simulink model "FDScanningTool"  (R2022b)
settings: Solver=ode1  StartTime=0.0  StopTime=Tobs  FixedStep=delta_t  RelTol=1e-3
values from neighbouring files (symbols this model uses):
  C = 2*pi*Eo*inv(Rp)    [LineParameters.m]    (also in ParametrosAB.m = 2*pi*Epsilon*inv(P); exe_FDScanningTool.m = 0.001)
  delta_t = 10E-6    (= 1e-05)    [exe_FDScanningTool.m]
  dist_time = 1    [exe_FDScanningTool.m]
  dist_value_0 = Idist_value    (= 0.05)    [exe_FDScanningTool.m]
  dist_value_a = [Isignal_dist3(:,1),zeros(samples_window,1)]    [exe_FDScanningTool.m]
  dist_value_b = [Isignal_dist3(:,1),zeros(samples_window,1)]    [exe_FDScanningTool.m]
  dist_value_c = Isignal_dist3    [exe_FDScanningTool.m]
  dist_value_d = Idist_value    (= 0.05)    [exe_FDScanningTool.m]
  dist_value_n = 0.0    (= 0)    [exe_FDScanningTool.m]
  dist_value_p = 0.0    (= 0)    [exe_FDScanningTool.m]
  dist_value_q = 0.0    (= 0)    [exe_FDScanningTool.m]
  f0 = 50    [exe_FDScanningTool.m]    (also in multisine.m = fs/Ns)
  fd = fd0(n)    [exe_FDScanningTool.m]
  Ipeak = 1    [exe_FDScanningTool.m]
  L = 0.001    [exe_FDScanningTool.m]
  phi = (2/3)*pi    (= 2.09439510239)    [exe_FDScanningTool.m]
  R = cond1(:,6)    [LineParameters.m]    (also in exe_FDScanningTool.m = 0.01778)
  R_load = 1E-6    (= 1e-06)    [exe_FDScanningTool.m]
  Rsource = 1E-3    (= 0.001)    [exe_FDScanningTool.m]
  signal_type = 1    [exe_FDScanningTool.m]
  Vpeak = 1    [exe_FDScanningTool.m]
libraries: spsSeriesRLCBranchLib x21, spsControlledCurrentSourceLib x12, spsControlledVoltageSourceLib x12, spsThreePhaseVIMeasurementLib x10, spsThreePhaseSeriesRLCBranchLib x6, spsGroundLib x5, spsDistributedParametersLineFrequencyDependentLib x1, spspowerguiLib x1
(part 1 of 2)
settings Model: SimulationMode=accelerator  Creator=Luis Angel  LastModifiedBy=Luis Angel

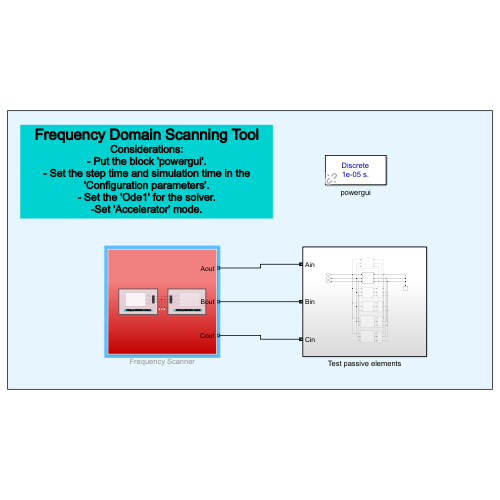
[thumbnail: Simulink's stored preview of the top-level diagram]
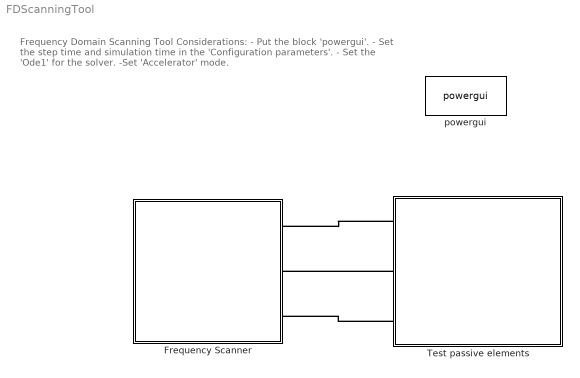
== system FDScanningTool ==
  note: Frequency Domain Scanning Tool
      | Considerations:
      | - Put the block 'powergui'.
      | - Set the step time and simulation time in the 'Configuration parameters'.
      | - Set the 'Ode1' for the solver.
      | -Set 'Accelerator' mode.
  Frequency Scanner : Subsystem
  Test passive elements : Subsystem
  powergui : spspowerguiLib/powergui  Priority=1  SimulationMode=Discrete  SampleTime=delta_t  frequency=60  Iterations=50  frequencyindice=0  Pbase=100e6  ErrMax=1e-4  UnitsV=kV  UnitsW=MW  buscounter=0  FunctionMessages=off  echomessages=off  EnableUseOfTLC=off  CurrentSourceSwitches=off  DisableSnubberDevices=off  DisableRonSwitches=off  DisableVfSwitches=off  DisplayEquations=off  AutomaticDiscreteSolvers=off  SolverType=Tustin/Backward Euler (TBE)  Interpol=off  ExternalGateDelay=off  methode=off  Ts=100  x0status=blocks  SPID=on  SwTol=0  HookPort=off  NonlinearTolerance=1e-4  nMaxIteration=100  ContinueOnMaxIteration=off  RestoreLinks=warning  ResistiveCurrentMeasurement=off  Frange=[0:2:500]  Ylog=off  Xlog=on  ShowGrid=off  save=off  variable=ZData  structure=0  ZoomFFT=off  StartTime=0.0  cycles=1  DisplayStyle=1  fundamental=60  FreqAxis=off  MaxFrequency=1000  frequencyindicesteady=1  RmsSteady=1  display=off
  connections:
  Test passive elements/LConn1 -- Frequency Scanner/RConn1
  Test passive elements/LConn2 -- Frequency Scanner/RConn2
  Test passive elements/LConn3 -- Frequency Scanner/RConn3

== system FDScanningTool/Frequency Scanner ==
  note: Current perturbation method
  note: Voltage perturbation method
  Current Strategy : Subsystem  Commented=on
  Three-Phase V-I Measurement1 : spsThreePhaseVIMeasurementLib/Three-Phase V-I Measurement  VoltageMeasurement=no  SetLabelV=on  LabelV=Vabc  Vpu=off  VpuLL=off  CurrentMeasurement=no  SetLabelI=on  LabelI=Iabc  Ipu=off  Pbase=100e6  Vbase=500e3  OutputType=Complex  PhasorSimulation=off  PSBequivalent=0
  Three-Phase V-I Measurement3 : spsThreePhaseVIMeasurementLib/Three-Phase V-I Measurement  VoltageMeasurement=no  SetLabelV=on  LabelV=Vabc  Vpu=off  VpuLL=off  CurrentMeasurement=no  SetLabelI=on  LabelI=Iabc  Ipu=off  Pbase=100e6  Vbase=500e3  OutputType=Complex  PhasorSimulation=off  PSBequivalent=0
  Voltage Strategy : Subsystem
  Aout : PMIOPort  Side=Right
  Bout : PMIOPort  Port=2  Side=Right
  Cout : PMIOPort  Port=3  Side=Right
  connections:
  Bout/RConn1 -- Three-Phase V-I Measurement3/RConn2 -- Three-Phase V-I Measurement1/RConn2
  Aout/RConn1 -- Three-Phase V-I Measurement3/RConn1 -- Three-Phase V-I Measurement1/RConn1
  Cout/RConn1 -- Three-Phase V-I Measurement1/RConn3 -- Three-Phase V-I Measurement3/RConn3
  Three-Phase V-I Measurement1/LConn1 -- Voltage Strategy/RConn1
  Three-Phase V-I Measurement1/LConn2 -- Voltage Strategy/RConn2
  Three-Phase V-I Measurement1/LConn3 -- Voltage Strategy/RConn3
  Three-Phase V-I Measurement3/LConn1 -- Current Strategy/LConn1
  Three-Phase V-I Measurement3/LConn2 -- Current Strategy/LConn2
  Three-Phase V-I Measurement3/LConn3 -- Current Strategy/LConn3

== system FDScanningTool/Test passive elements ==
  For the paper : spsDistributedParametersLineFrequencyDependentLib/Distributed Parameters Line (Frequency-Dependent)  Commented=on  WBfile=Line_735kV.mat  L=100  NbPhases=3  Frange=1.00e-02 Hz to 1.00e+05 Hz, 141 points.  Comments=|  Measurements=None
      | Example of a 735 KV three-phase line
      |
      | Three bundles of 4 Bersfort ACSR 1355 MCM conductors
      | Two 1/2 inch diameter steel grounds wires
      |
      | Ytower =Ymin =  average heights of conductors
      settings: LibrarySourceBlock=|
      | sps_lib/Power Grid Elements/Distributed Parameters Line
      | (Frequency-Dependent)
  Ground17 : spsGroundLib/Ground  LConnTagsString=a
  TL PI Asymmetrical : Subsystem  Commented=on
  TL PI Symmetrical : Subsystem  Commented=on
  Three-Phase Series RLC Branch1 : spsThreePhaseSeriesRLCBranchLib/Three-Phase Series RLC Branch  LConnTagsString=A|B|C  RConnTagsString=A|B|C  BranchType=RLC  Resistance=R  Inductance=L  Capacitance=C  Measurements=None
  Three-Phase Series RLC Branch11 : spsThreePhaseSeriesRLCBranchLib/Three-Phase Series RLC Branch  Commented=on  LConnTagsString=A|B|C  RConnTagsString=A|B|C  BranchType=R  Resistance=R_load  Inductance=1e-3  Capacitance=1e-6  Measurements=None
  Three-Phase Series RLC Branch12 : spsThreePhaseSeriesRLCBranchLib/Three-Phase Series RLC Branch  Commented=on  LConnTagsString=A|B|C  RConnTagsString=A|B|C  BranchType=R  Resistance=R_load  Inductance=1e-3  Capacitance=1e-6  Measurements=None
  Three-Phase Series RLC Branch2 : spsThreePhaseSeriesRLCBranchLib/Three-Phase Series RLC Branch  Commented=on  LConnTagsString=A|B|C  RConnTagsString=A|B|C  BranchType=R  Resistance=R_load  Inductance=1e-3  Capacitance=1e-6  Measurements=None
  Unbalanced RLC2 : Subsystem  Commented=on
  Ain : PMIOPort  Side=Left
  Bin : PMIOPort  Port=2  Side=Left
  Cin : PMIOPort  Port=3  Side=Left
  connections:
  TL PI Symmetrical/RConn1 -- Three-Phase Series RLC Branch11/LConn1
  Three-Phase Series RLC Branch12/LConn1 -- TL PI Asymmetrical/RConn1
  TL PI Symmetrical/LConn3 -- For the paper/LConn3 -- TL PI Asymmetrical/LConn3 -- Cin/RConn1 -- Unbalanced RLC2/LConn3 -- Three-Phase Series RLC Branch1/LConn3
  TL PI Asymmetrical/LConn1 -- For the paper/LConn1 -- Unbalanced RLC2/LConn1 -- Ain/RConn1 -- Three-Phase Series RLC Branch1/LConn1 -- TL PI Symmetrical/LConn1
  Three-Phase Series RLC Branch12/LConn2 -- TL PI Asymmetrical/RConn2
  Unbalanced RLC2/LConn2 -- For the paper/LConn2 -- TL PI Asymmetrical/LConn2 -- TL PI Symmetrical/LConn2 -- Bin/RConn1 -- Three-Phase Series RLC Branch1/LConn2
  TL PI Symmetrical/RConn2 -- Three-Phase Series RLC Branch11/LConn2
  Three-Phase Series RLC Branch12/LConn3 -- TL PI Asymmetrical/RConn3
  TL PI Symmetrical/RConn3 -- Three-Phase Series RLC Branch11/LConn3
  Three-Phase Series RLC Branch1/RConn2 -- Unbalanced RLC2/RConn2 -- Unbalanced RLC2/RConn3 -- Three-Phase Series RLC Branch1/RConn3 -- Three-Phase Series RLC Branch2/RConn3 -- Three-Phase Series RLC Branch12/RConn3 -- Three-Phase Series RLC Branch11/RConn3 -- Ground17/LConn1 -- Three-Phase Series RLC Branch2/RConn1 -- Three-Phase Series RLC Branch12/RConn1 -- Three-Phase Series RLC Branch11/RConn1 -- Unbalanced RLC2/RConn1 -- Three-Phase Series RLC Branch1/RConn1 -- Three-Phase Series RLC Branch2/RConn2 -- Three-Phase Series RLC Branch12/RConn2 -- Three-Phase Series RLC Branch11/RConn2
  For the paper/RConn1 -- Three-Phase Series RLC Branch2/LConn1
  For the paper/RConn2 -- Three-Phase Series RLC Branch2/LConn2
  For the paper/RConn3 -- Three-Phase Series RLC Branch2/LConn3

== system FDScanningTool/Frequency Scanner/Current Strategy ==
  note: qd0 scan
  note: Fundamental source
  note: pn0 scan
  note: ABC scan
  ABCdisturbance2 : Subsystem  Commented=on
  Current Fundamental Source : Subsystem
      settings: PortSchema="{\"entries\":[{\"content\":{\"sides\":[{\"content\":{\"connectorIds\":[\"Out1\"]},\"type\":\"ConnectorPlacement.EquallySpacedRectSide\",\"uuid\":\"2a4baa29-0316-4256-b4e1-e3ef1d370b3b\"},{\"content\":{\"connectorIds\":[\"RConn1\",\"RConn2\",\"RConn3\"],\"side\":\"RIGHT\"},\"type\":\"ConnectorPlacement.EquallySpacedRectSide\",\"uuid\":\"3108b85a-ac52-49ed-83a6-d77923640585\"},{\"content\":{\"connectorIds\":[],\"side\":\"TOP\"},\"type\":\"ConnectorPlacement.EquallySpacedRectSide\",\"uuid\":\"4093502e-3b8b-4232-aa57-5a461ca3ca63\"},{\"content\":{\"connectorIds\":[\"RConn4\"],\"side\":\"BOTTOM\"},\"type\":\"ConnectorPlacement.EquallySpacedRectSide\",\"uuid\":\"50c06102-7582-4746-a571-3f791f943454\"}]},\"type\":\"ConnectorPlacement.EquallySpacedConnector\",\"uuid\":\"209f4db4-fe77-48a5-84ae-6773984a343b\"}],\"packageUris\":[\"http://schema.mathworks.com/mf0/Connector/R2020b\"],\"version\":\"1.0\"}"
  Three-Phase V-I Measurement2 : spsThreePhaseVIMeasurementLib/Three-Phase V-I Measurement  VoltageMeasurement=no  SetLabelV=on  LabelV=Vabc  Vpu=off  VpuLL=off  CurrentMeasurement=no  SetLabelI=on  LabelI=Iabc  Ipu=off  Pbase=100e6  Vbase=500e3  OutputType=Complex  PhasorSimulation=off  PSBequivalent=0
  pn0disturbance2 : Subsystem
  qd0disturbance2 : Subsystem  Commented=on
      settings: PortSchema="{\"entries\":[{\"content\":{\"sides\":[{\"content\":{\"connectorIds\":[\"LConn1\",\"LConn2\",\"LConn3\",\"LConn4\"]},\"type\":\"ConnectorPlacement.EquallySpacedRectSide\",\"uuid\":\"96b61a08-e73c-4bf9-b44c-8e6d57b8ef4a\"},{\"content\":{\"connectorIds\":[\"RConn1\",\"RConn2\",\"RConn3\"],\"side\":\"RIGHT\"},\"type\":\"ConnectorPlacement.EquallySpacedRectSide\",\"uuid\":\"3a0e4222-9b60-4a58-9d08-3b159ebff1b9\"},{\"content\":{\"connectorIds\":[\"In1\"],\"side\":\"TOP\"},\"type\":\"ConnectorPlacement.EquallySpacedRectSide\",\"uuid\":\"61af63da-f353-4270-b8c9-89c35459604e\"}]},\"type\":\"ConnectorPlacement.EquallySpacedConnector\",\"uuid\":\"24d596f4-e3d4-42a2-b524-8b1140a91bdb\"}],\"packageUris\":[\"http://schema.mathworks.com/mf0/Connector/R2020b\"],\"version\":\"1.0\"}"
  Aout : PMIOPort  Side=Left
  Bout : PMIOPort  Port=2  Side=Left
  Cout : PMIOPort  Port=3  Side=Left
  wires:
  [theta] -> qd0disturbance2/1(theta)
  Current Fundamental Source/1(theta) -> [theta]
  connections:
  pn0disturbance2/RConn1 -- Aout/RConn1 -- ABCdisturbance2/RConn1 -- qd0disturbance2/RConn1
  pn0disturbance2/RConn2 -- Bout/RConn1 -- ABCdisturbance2/RConn2 -- qd0disturbance2/RConn2
  Current Fundamental Source/RConn2 -- Three-Phase V-I Measurement2/LConn2
  Three-Phase V-I Measurement2/RConn2 -- pn0disturbance2/LConn2 -- ABCdisturbance2/LConn2 -- qd0disturbance2/LConn2
  Current Fundamental Source/RConn3 -- Three-Phase V-I Measurement2/LConn3
  pn0disturbance2/RConn3 -- Cout/RConn1 -- ABCdisturbance2/RConn3 -- qd0disturbance2/RConn3
  Three-Phase V-I Measurement2/RConn1 -- pn0disturbance2/LConn1 -- ABCdisturbance2/LConn1 -- qd0disturbance2/LConn1
  Current Fundamental Source/RConn4 -- pn0disturbance2/LConn4 -- ABCdisturbance2/LConn4 -- qd0disturbance2/LConn4
  Three-Phase V-I Measurement2/RConn3 -- pn0disturbance2/LConn3 -- ABCdisturbance2/LConn3 -- qd0disturbance2/LConn3
  Current Fundamental Source/RConn1 -- Three-Phase V-I Measurement2/LConn1

== system FDScanningTool/Frequency Scanner/Voltage Strategy ==
  note: Fundamental source
  note: pn0 scan
  note: ABC scan
  note: qd0 scan
  ABCdisturbance : Subsystem  Commented=on
  Three-Phase V-I Measurement : spsThreePhaseVIMeasurementLib/Three-Phase V-I Measurement  VoltageMeasurement=no  SetLabelV=on  LabelV=Vabc  Vpu=off  VpuLL=off  CurrentMeasurement=no  SetLabelI=on  LabelI=Iabc  Ipu=off  Pbase=100e6  Vbase=500e3  OutputType=Complex  PhasorSimulation=off  PSBequivalent=0
  Voltage Fundamental Source : Subsystem
      settings: PortSchema="{\"entries\":[{\"content\":{\"sides\":[{\"content\":{\"connectorIds\":[\"Out1\"]},\"type\":\"ConnectorPlacement.EquallySpacedRectSide\",\"uuid\":\"3dbf8d23-22ab-4ddc-ae4a-19197e180312\"},{\"content\":{\"connectorIds\":[\"RConn1\",\"RConn2\",\"RConn3\"],\"side\":\"RIGHT\"},\"type\":\"ConnectorPlacement.EquallySpacedRectSide\",\"uuid\":\"df914263-db35-4888-aa99-5dec7a54c6e0\"},{\"content\":{\"connectorIds\":[],\"side\":\"TOP\"},\"type\":\"ConnectorPlacement.EquallySpacedRectSide\",\"uuid\":\"815bd59d-9d4f-4637-8c0a-95368e7d07f9\"}]},\"type\":\"ConnectorPlacement.EquallySpacedConnector\",\"uuid\":\"b7ffca83-a6f6-4340-8cfa-6aec16cec0d1\"}],\"packageUris\":[\"http://schema.mathworks.com/mf0/Connector/R2020b\"],\"version\":\"1.0\"}"
  pn0disturbance : Subsystem
  qd0disturbance : Subsystem  Commented=on
      settings: PortSchema="{\"entries\":[{\"content\":{\"sides\":[{\"content\":{\"connectorIds\":[\"LConn1\",\"LConn2\",\"LConn3\"]},\"type\":\"ConnectorPlacement.EquallySpacedRectSide\",\"uuid\":\"96b61a08-e73c-4bf9-b44c-8e6d57b8ef4a\"},{\"content\":{\"connectorIds\":[\"RConn1\",\"RConn2\",\"RConn3\"],\"side\":\"RIGHT\"},\"type\":\"ConnectorPlacement.EquallySpacedRectSide\",\"uuid\":\"3a0e4222-9b60-4a58-9d08-3b159ebff1b9\"},{\"content\":{\"connectorIds\":[\"In1\"],\"side\":\"TOP\"},\"type\":\"ConnectorPlacement.EquallySpacedRectSide\",\"uuid\":\"61af63da-f353-4270-b8c9-89c35459604e\"}]},\"type\":\"ConnectorPlacement.EquallySpacedConnector\",\"uuid\":\"24d596f4-e3d4-42a2-b524-8b1140a91bdb\"}],\"packageUris\":[\"http://schema.mathworks.com/mf0/Connector/R2020b\"],\"version\":\"1.0\"}"
  Aout : PMIOPort  Side=Right
  Bout : PMIOPort  Port=2  Side=Right
  Cout : PMIOPort  Port=3  Side=Right
  wires:
  Voltage Fundamental Source/1(theta) -> [theta]
  [theta] -> qd0disturbance/1(theta)
  connections:
  ABCdisturbance/RConn2 -- Bout/RConn1 -- pn0disturbance/RConn2 -- qd0disturbance/RConn2
  Voltage Fundamental Source/RConn1 -- Three-Phase V-I Measurement/LConn1
  qd0disturbance/LConn3 -- ABCdisturbance/LConn3 -- Three-Phase V-I Measurement/RConn3 -- pn0disturbance/LConn3
  ABCdisturbance/RConn1 -- Aout/RConn1 -- pn0disturbance/RConn1 -- qd0disturbance/RConn1
  Voltage Fundamental Source/RConn2 -- Three-Phase V-I Measurement/LConn2
  Voltage Fundamental Source/RConn3 -- Three-Phase V-I Measurement/LConn3
  ABCdisturbance/RConn3 -- Cout/RConn1 -- pn0disturbance/RConn3 -- qd0disturbance/RConn3
  qd0disturbance/LConn1 -- ABCdisturbance/LConn1 -- Three-Phase V-I Measurement/RConn1 -- pn0disturbance/LConn1
  qd0disturbance/LConn2 -- ABCdisturbance/LConn2 -- Three-Phase V-I Measurement/RConn2 -- pn0disturbance/LConn2

== system FDScanningTool/Test passive elements/TL PI Asymmetrical ==
  Ground6 : spsGroundLib/Ground  LConnTagsString=a
  Series RLC Branch1 : spsSeriesRLCBranchLib/Series RLC Branch  LConnTagsString=__new0  RConnTagsString=__new0  BranchType=RL  Resistance=R*0.9  Inductance=L*0.9  SetiL0=off  InitialCurrent=0  Capacitance=1e-6  Setx0=off  InitialVoltage=0  Measurements=None
  Series RLC Branch2 : spsSeriesRLCBranchLib/Series RLC Branch  LConnTagsString=__new0  RConnTagsString=__new0  BranchType=C  Resistance=1  Inductance=1e-3  SetiL0=off  InitialCurrent=0  Capacitance=C*0.9/2  Setx0=off  InitialVoltage=Vinit  Measurements=None
  Series RLC Branch3 : spsSeriesRLCBranchLib/Series RLC Branch  LConnTagsString=__new0  RConnTagsString=__new0  BranchType=RL  Resistance=R  Inductance=L  SetiL0=off  InitialCurrent=0  Capacitance=1e-6  Setx0=off  InitialVoltage=0  Measurements=None
  Series RLC Branch4 : spsSeriesRLCBranchLib/Series RLC Branch  LConnTagsString=__new0  RConnTagsString=__new0  BranchType=C  Resistance=1  Inductance=1e-3  SetiL0=off  InitialCurrent=0  Capacitance=C/2  Setx0=off  InitialVoltage=Vinit  Measurements=None
  Series RLC Branch5 : spsSeriesRLCBranchLib/Series RLC Branch  LConnTagsString=__new0  RConnTagsString=__new0  BranchType=C  Resistance=1  Inductance=1e-3  SetiL0=off  InitialCurrent=0  Capacitance=C/2  Setx0=off  InitialVoltage=Vinit  Measurements=None
  Series RLC Branch6 : spsSeriesRLCBranchLib/Series RLC Branch  LConnTagsString=__new0  RConnTagsString=__new0  BranchType=C  Resistance=1  Inductance=1e-3  SetiL0=off  InitialCurrent=0  Capacitance=C*0.9/2  Setx0=off  InitialVoltage=Vinit  Measurements=None
  Series RLC Branch7 : spsSeriesRLCBranchLib/Series RLC Branch  LConnTagsString=__new0  RConnTagsString=__new0  BranchType=RL  Resistance=R*0.8  Inductance=L*0.8  SetiL0=off  InitialCurrent=0  Capacitance=1e-6  Setx0=off  InitialVoltage=0  Measurements=None
  Series RLC Branch8 : spsSeriesRLCBranchLib/Series RLC Branch  LConnTagsString=__new0  RConnTagsString=__new0  BranchType=C  Resistance=1  Inductance=1e-3  SetiL0=off  InitialCurrent=0  Capacitance=C*0.8/2  Setx0=off  InitialVoltage=Vinit  Measurements=None
  Series RLC Branch9 : spsSeriesRLCBranchLib/Series RLC Branch  LConnTagsString=__new0  RConnTagsString=__new0  BranchType=C  Resistance=1  Inductance=1e-3  SetiL0=off  InitialCurrent=0  Capacitance=C*0.8/2  Setx0=off  InitialVoltage=Vinit  Measurements=None
  A : PMIOPort  Side=Left
  B : PMIOPort  Port=2  Side=Left
  C : PMIOPort  Port=3  Side=Left
  a : PMIOPort  Port=4  Side=Right
  b : PMIOPort  Port=5  Side=Right
  c : PMIOPort  Port=6  Side=Right
  connections:
  Series RLC Branch5/LConn1 -- a/RConn1 -- Series RLC Branch3/RConn1
  Series RLC Branch2/RConn1 -- Series RLC Branch6/RConn1 -- Series RLC Branch8/RConn1 -- Series RLC Branch9/RConn1 -- Ground6/LConn1 -- Series RLC Branch5/RConn1 -- Series RLC Branch4/RConn1
  Series RLC Branch3/LConn1 -- A/RConn1 -- Series RLC Branch4/LConn1
  Series RLC Branch1/LConn1 -- Series RLC Branch2/LConn1 -- B/RConn1
  Series RLC Branch6/LConn1 -- Series RLC Branch1/RConn1 -- b/RConn1
  Series RLC Branch7/LConn1 -- Series RLC Branch8/LConn1 -- C/RConn1
  Series RLC Branch9/LConn1 -- Series RLC Branch7/RConn1 -- c/RConn1

== system FDScanningTool/Test passive elements/TL PI Symmetrical ==
  Ground3 : spsGroundLib/Ground  LConnTagsString=a
  Series RLC Branch1 : spsSeriesRLCBranchLib/Series RLC Branch  LConnTagsString=__new0  RConnTagsString=__new0  BranchType=RL  Resistance=R  Inductance=L  SetiL0=off  InitialCurrent=0  Capacitance=1e-6  Setx0=off  InitialVoltage=0  Measurements=None
  Series RLC Branch{2,4..6,8..9} (6 alike) : spsSeriesRLCBranchLib/Series RLC Branch  LConnTagsString=__new0  RConnTagsString=__new0  BranchType=C  Resistance=1  Inductance=1e-3  SetiL0=off  InitialCurrent=0  Capacitance=C/2  Setx0=off  InitialVoltage=Vinit  Measurements=None
  Series RLC Branch3 : spsSeriesRLCBranchLib/Series RLC Branch  LConnTagsString=__new0  RConnTagsString=__new0  BranchType=RL  Resistance=R  Inductance=L  SetiL0=off  InitialCurrent=0  Capacitance=1e-6  Setx0=off  InitialVoltage=0  Measurements=None
  Series RLC Branch7 : spsSeriesRLCBranchLib/Series RLC Branch  LConnTagsString=__new0  RConnTagsString=__new0  BranchType=RL  Resistance=R  Inductance=L  SetiL0=off  InitialCurrent=0  Capacitance=1e-6  Setx0=off  InitialVoltage=0  Measurements=None
  A : PMIOPort  Side=Left
  B : PMIOPort  Port=2  Side=Left
  C : PMIOPort  Port=3  Side=Left
  a : PMIOPort  Port=4  Side=Right
  b : PMIOPort  Port=5  Side=Right
  c : PMIOPort  Port=6  Side=Right
  connections:
  Series RLC Branch5/LConn1 -- a/RConn1 -- Series RLC Branch3/RConn1
  Series RLC Branch3/LConn1 -- A/RConn1 -- Series RLC Branch4/LConn1
  Series RLC Branch1/LConn1 -- Series RLC Branch2/LConn1 -- B/RConn1
  Series RLC Branch6/LConn1 -- Series RLC Branch1/RConn1 -- b/RConn1
  Series RLC Branch6/RConn1 -- Series RLC Branch8/RConn1 -- Series RLC Branch9/RConn1 -- Series RLC Branch4/RConn1 -- Series RLC Branch5/RConn1 -- Ground3/LConn1 -- Series RLC Branch2/RConn1
  Series RLC Branch7/LConn1 -- Series RLC Branch8/LConn1 -- C/RConn1
  Series RLC Branch9/LConn1 -- Series RLC Branch7/RConn1 -- c/RConn1

== system FDScanningTool/Test passive elements/Unbalanced RLC2 ==
  Series RLC Branch : spsSeriesRLCBranchLib/Series RLC Branch  LConnTagsString=__new0  RConnTagsString=__new0  BranchType=RLC  Resistance=R  Inductance=L  SetiL0=off  InitialCurrent=0  Capacitance=C  Setx0=off  InitialVoltage=0  Measurements=None
  Series RLC Branch1 : spsSeriesRLCBranchLib/Series RLC Branch  LConnTagsString=__new0  RConnTagsString=__new0  BranchType=RLC  Resistance=R*0.9  Inductance=L*0.9  SetiL0=off  InitialCurrent=0  Capacitance=C*0.9  Setx0=off  InitialVoltage=0  Measurements=None
  Series RLC Branch2 : spsSeriesRLCBranchLib/Series RLC Branch  LConnTagsString=__new0  RConnTagsString=__new0  BranchType=RLC  Resistance=R*0.8  Inductance=L*0.8  SetiL0=off  InitialCurrent=0  Capacitance=C*0.8  Setx0=off  InitialVoltage=0  Measurements=None
  Conn1 : PMIOPort  Side=Left
  Conn2 : PMIOPort  Port=2  Side=Right
  Conn3 : PMIOPort  Port=3  Side=Left
  Conn4 : PMIOPort  Port=4  Side=Right
  Conn5 : PMIOPort  Port=5  Side=Left
  Conn6 : PMIOPort  Port=6  Side=Right
  connections:
  Series RLC Branch/LConn1 -- Conn1/RConn1
  Series RLC Branch2/RConn1 -- Conn6/RConn1
  Series RLC Branch1/RConn1 -- Conn4/RConn1
  Series RLC Branch2/LConn1 -- Conn5/RConn1
  Series RLC Branch1/LConn1 -- Conn3/RConn1
  Series RLC Branch/RConn1 -- Conn2/RConn1

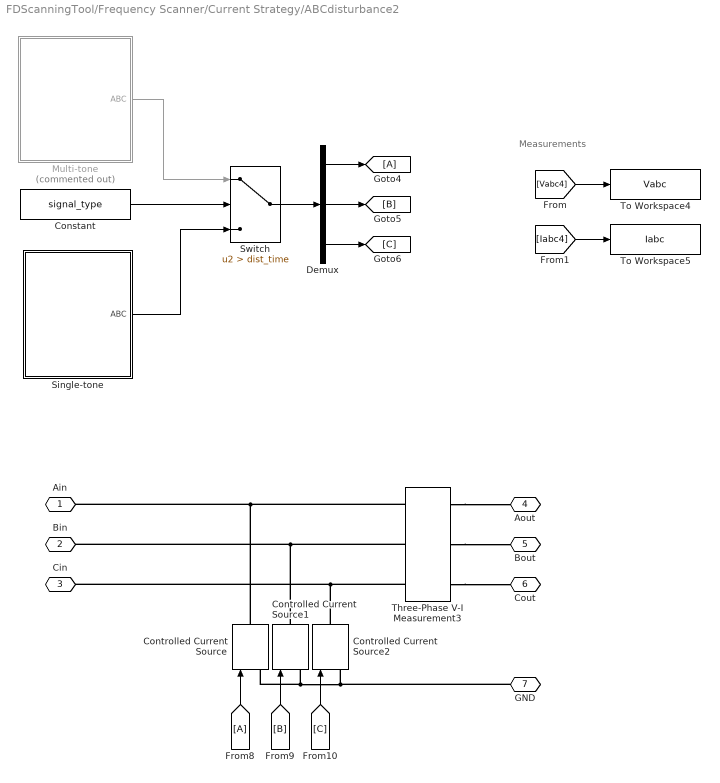
== system FDScanningTool/Frequency Scanner/Current Strategy/ABCdisturbance2 ==
  note: Measurements
  Constant : Constant  Value=signal_type
  Controlled Current Source : spsControlledCurrentSourceLib/Controlled Current Source  Initialize=off  Source_Type=AC  Amplitude=0  Phase=0  Frequency=0  Measurements=None
  Controlled Current Source1 : spsControlledCurrentSourceLib/Controlled Current Source  Initialize=off  Source_Type=AC  Amplitude=0  Phase=0  Frequency=0  Measurements=None
  Controlled Current Source2 : spsControlledCurrentSourceLib/Controlled Current Source  Initialize=off  Source_Type=AC  Amplitude=0  Phase=0  Frequency=0  Measurements=None
  Demux : Demux  Outputs=3
  From8 : From
  Goto4 : Goto
  Multi-tone : Subsystem  Commented=on
  Single-tone : Subsystem
  Switch : Switch  Criteria=u2 > Threshold  Threshold=dist_time  SaturateOnIntegerOverflow=off  InputSameDT=off
  Three-Phase V-I Measurement3 : spsThreePhaseVIMeasurementLib/Three-Phase V-I Measurement  VoltageMeasurement=phase-to-ground  SetLabelV=on  LabelV=Vabc4  Vpu=off  VpuLL=off  CurrentMeasurement=yes  SetLabelI=on  LabelI=Iabc4  Ipu=off  Pbase=100e6  Vbase=500e3  OutputType=Complex  PhasorSimulation=off  PSBequivalent=0
  To Workspace4 : ToWorkspace  VariableName=Vabc  SampleTime=-1
  To Workspace5 : ToWorkspace  VariableName=Iabc  SampleTime=-1
  Ain : PMIOPort  Side=Left
  Bin : PMIOPort  Port=2  Side=Left
  Cin : PMIOPort  Port=3  Side=Left
  Aout : PMIOPort  Port=4  Side=Right
  Bout : PMIOPort  Port=5  Side=Right
  Cout : PMIOPort  Port=6  Side=Right
  GND : PMIOPort  Port=7  Side=Left
  wires:
  [Vabc4] -> To Workspace4/1
  [Iabc4] -> To Workspace5/1
  [C] -> Controlled Current Source2/1
  [B] -> Controlled Current Source1/1
  From8/1 -> Controlled Current Source/1
  Constant/1 -> Switch/2
  Multi-tone/1(ABC) -> Switch/1
  Demux/1 -> Goto4/1
  Demux/2 -> [B]
  Demux/3 -> [C]
  Switch/1 -> Demux/1
  Single-tone/1(ABC) -> Switch/3
  connections:
  Controlled Current Source1/LConn1 -- GND/RConn1 -- Controlled Current Source2/LConn1 -- Controlled Current Source/LConn1
  Controlled Current Source/RConn1 -- Three-Phase V-I Measurement3/LConn1 -- Ain/RConn1
  Controlled Current Source2/RConn1 -- Three-Phase V-I Measurement3/LConn3 -- Cin/RConn1
  Controlled Current Source1/RConn1 -- Three-Phase V-I Measurement3/LConn2 -- Bin/RConn1
  Three-Phase V-I Measurement3/RConn1 -- Aout/RConn1
  Three-Phase V-I Measurement3/RConn2 -- Bout/RConn1
  Three-Phase V-I Measurement3/RConn3 -- Cout/RConn1

== system FDScanningTool/Frequency Scanner/Current Strategy/Current Fundamental Source ==
  Controlled Current Source : spsControlledCurrentSourceLib/Controlled Current Source  Initialize=off  Source_Type=AC  Amplitude=0  Phase=0  Frequency=0  Measurements=None
  Controlled Current Source1 : spsControlledCurrentSourceLib/Controlled Current Source  Initialize=off  Source_Type=AC  Amplitude=0  Phase=0  Frequency=0  Measurements=None
  Controlled Current Source2 : spsControlledCurrentSourceLib/Controlled Current Source  Initialize=off  Source_Type=AC  Amplitude=0  Phase=0  Frequency=0  Measurements=None
  Grid Voltages1 : Subsystem
  Ground : spsGroundLib/Ground  LConnTagsString=a
  Three-Phase Series RLC Branch : spsThreePhaseSeriesRLCBranchLib/Three-Phase Series RLC Branch  LConnTagsString=A|B|C  RConnTagsString=A|B|C  BranchType=R  Resistance=1/Rsource  Inductance=1e-3  Capacitance=1e-6  Measurements=None
  VzA : PMIOPort  Side=Right
  VzB : PMIOPort  Port=2  Side=Right
  VzC : PMIOPort  Port=3  Side=Right
  GND : PMIOPort  Port=4  Side=Right
  theta : Outport
  wires:
  Grid Voltages1/3(VC) -> Controlled Current Source/1
  Grid Voltages1/2(VB) -> Controlled Current Source1/1
  Grid Voltages1/1(VA) -> Controlled Current Source2/1
  Grid Voltages1/4(theta) -> theta/1
  connections:
  Controlled Current Source2/RConn1 -- Three-Phase Series RLC Branch/LConn1 -- VzA/RConn1
  Controlled Current Source1/RConn1 -- Three-Phase Series RLC Branch/LConn2 -- VzB/RConn1
  Controlled Current Source/RConn1 -- Three-Phase Series RLC Branch/LConn3 -- VzC/RConn1
  Ground/LConn1 -- Controlled Current Source/LConn1 -- Controlled Current Source1/LConn1 -- Controlled Current Source2/LConn1 -- Three-Phase Series RLC Branch/RConn3 -- Three-Phase Series RLC Branch/RConn2 -- Three-Phase Series RLC Branch/RConn1 -- GND/RConn1

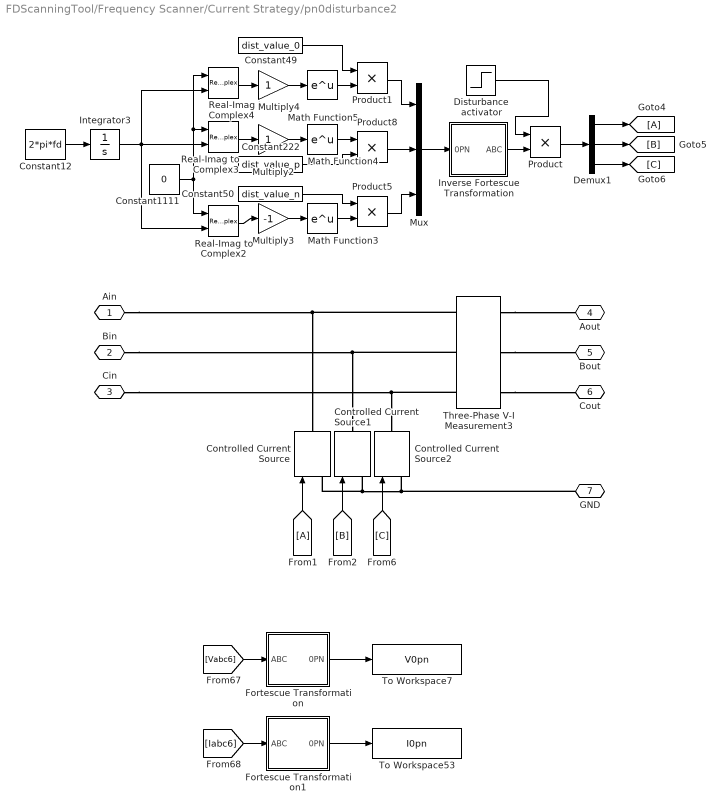
== system FDScanningTool/Frequency Scanner/Current Strategy/pn0disturbance2 ==
  Constant1111 : Constant  Value=0
  Constant12 : Constant  Value=2*pi*fd  SampleTime=delta_t
  Constant222 : Constant  Value=dist_value_p
  Constant49 : Constant  Value=dist_value_0
  Constant50 : Constant  Value=dist_value_n
  Controlled Current Source : spsControlledCurrentSourceLib/Controlled Current Source  Initialize=off  Source_Type=AC  Amplitude=0  Phase=0  Frequency=0  Measurements=None
  Controlled Current Source1 : spsControlledCurrentSourceLib/Controlled Current Source  Initialize=off  Source_Type=AC  Amplitude=0  Phase=0  Frequency=0  Measurements=None
  Controlled Current Source2 : spsControlledCurrentSourceLib/Controlled Current Source  Initialize=off  Source_Type=AC  Amplitude=0  Phase=0  Frequency=0  Measurements=None
  Demux1 : Demux  Outputs=3
  Disturbance activator : Step  Time=dist_time  SampleTime=delta_t
  Fortescue Transformation : Subsystem
  Fortescue Transformation1 : Subsystem
  From1 : From
  Goto4 : Goto
  Integrator3 : Integrator
  Inverse Fortescue Transformation : Subsystem
  Math Function3 : Math
  Math Function4 : Math
  Math Function5 : Math
  Multiply2 : Gain
  Multiply3 : Gain  Gain=-1
  Multiply4 : Gain
  Mux : Mux  Inputs=3
  Product{,1,5,8} (4 alike) : Product
  Real-Imag to Complex2 : RealImagToComplex
  Real-Imag to Complex3 : RealImagToComplex
  Real-Imag to Complex4 : RealImagToComplex
  Three-Phase V-I Measurement3 : spsThreePhaseVIMeasurementLib/Three-Phase V-I Measurement  VoltageMeasurement=phase-to-ground  SetLabelV=on  LabelV=Vabc6  Vpu=off  VpuLL=off  CurrentMeasurement=yes  SetLabelI=on  LabelI=Iabc6  Ipu=off  Pbase=100e6  Vbase=500e3  OutputType=Complex  PhasorSimulation=off  PSBequivalent=0
  To Workspace53 : ToWorkspace  VariableName=I0pn  SampleTime=-1
  To Workspace7 : ToWorkspace  VariableName=V0pn  SampleTime=-1
  Ain : PMIOPort  Side=Left
  Bin : PMIOPort  Port=2  Side=Left
  Cin : PMIOPort  Port=3  Side=Left
  Aout : PMIOPort  Port=4  Side=Right
  Bout : PMIOPort  Port=5  Side=Right
  Cout : PMIOPort  Port=6  Side=Right
  GND : PMIOPort  Port=7  Side=Left
  wires:
  Product/1 -> Demux1/1
  Demux1/1 -> Goto4/1
  Demux1/3 -> [C]
  Demux1/2 -> [B]
  Mux/1 -> Inverse Fortescue Transformation/1(0PN)
  Multiply2/1 -> Math Function4/1
  Integrator3/1 -> Real-Imag to Complex2/2, Real-Imag to Complex3/2, Real-Imag to Complex4/2
  Constant1111/1 -> Real-Imag to Complex4/1, Real-Imag to Complex3/1, Real-Imag to Complex2/1
  Real-Imag to Complex3/1 -> Multiply2/1
  Multiply3/1 -> Math Function3/1
  Constant12/1 -> Integrator3/1
  Real-Imag to Complex2/1 -> Multiply3/1
  Math Function5/1 -> Product1/2
  Real-Imag to Complex4/1 -> Multiply4/1
  Multiply4/1 -> Math Function5/1
  Product1/1 -> Mux/1
  Disturbance activator/1 -> Product/1
  Inverse Fortescue Transformation/1(ABC) -> Product/2
  Constant49/1 -> Product1/1
  Math Function3/1 -> Product5/2
  Constant50/1 -> Product5/1
  Math Function4/1 -> Product8/1
  Constant222/1 -> Product8/2
  Product8/1 -> Mux/2
  Product5/1 -> Mux/3
  [Vabc6] -> Fortescue Transformation/1(ABC)
  [Iabc6] -> Fortescue Transformation1/1(ABC)
  Fortescue Transformation/1(0PN) -> To Workspace7/1
  Fortescue Transformation1/1(0PN) -> To Workspace53/1
  [B] -> Controlled Current Source1/1
  [C] -> Controlled Current Source2/1
  From1/1 -> Controlled Current Source/1
  connections:
  Cin/RConn1 -- Three-Phase V-I Measurement3/LConn3 -- Controlled Current Source2/RConn1
  Controlled Current Source1/LConn1 -- GND/RConn1 -- Controlled Current Source2/LConn1 -- Controlled Current Source/LConn1
  Ain/RConn1 -- Three-Phase V-I Measurement3/LConn1 -- Controlled Current Source/RConn1
  Bin/RConn1 -- Three-Phase V-I Measurement3/LConn2 -- Controlled Current Source1/RConn1
  Three-Phase V-I Measurement3/RConn3 -- Cout/RConn1
  Three-Phase V-I Measurement3/RConn2 -- Bout/RConn1
  Three-Phase V-I Measurement3/RConn1 -- Aout/RConn1

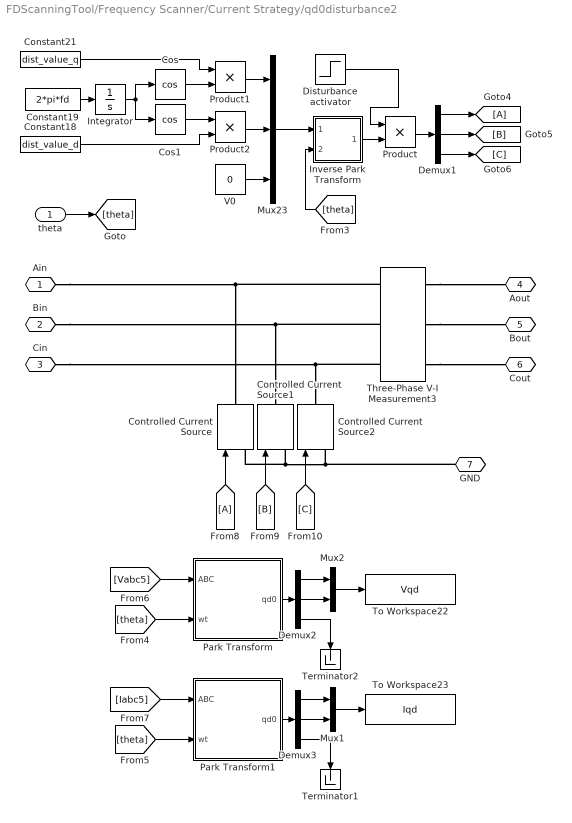
== system FDScanningTool/Frequency Scanner/Current Strategy/qd0disturbance2 ==
  theta : Inport
  Constant18 : Constant  Value=dist_value_d
  Constant19 : Constant  Value=2*pi*fd
  Constant21 : Constant  Value=dist_value_q
  Controlled Current Source : spsControlledCurrentSourceLib/Controlled Current Source  Initialize=off  Source_Type=AC  Amplitude=0  Phase=0  Frequency=0  Measurements=None
  Controlled Current Source1 : spsControlledCurrentSourceLib/Controlled Current Source  Initialize=off  Source_Type=AC  Amplitude=0  Phase=0  Frequency=0  Measurements=None
  Controlled Current Source2 : spsControlledCurrentSourceLib/Controlled Current Source  Initialize=off  Source_Type=AC  Amplitude=0  Phase=0  Frequency=0  Measurements=None
  Cos : Trigonometry  Operator=cos
  Cos1 : Trigonometry  Operator=cos
  Demux1 : Demux  Outputs=3
  Demux2 : Demux  Outputs=3
  Demux3 : Demux  Outputs=3
  Disturbance activator : Step  Time=dist_time  Before=0.0  After=1.0  SampleTime=delta_t
  From8 : From
  Goto4 : Goto
  Integrator : Integrator
  Inverse Park Transform : Subsystem
  Mux1 : Mux  Inputs=2
  Mux2 : Mux  Inputs=2
  Mux23 : Mux  Inputs=3
  Park Transform : Subsystem
  Park Transform1 : Subsystem
  Product : Product
  Product1 : Product
  Product2 : Product
  Terminator1 : Terminator
  Terminator2 : Terminator
  Three-Phase V-I Measurement3 : spsThreePhaseVIMeasurementLib/Three-Phase V-I Measurement  VoltageMeasurement=phase-to-ground  SetLabelV=on  LabelV=Vabc5  Vpu=off  VpuLL=off  CurrentMeasurement=yes  SetLabelI=on  LabelI=Iabc5  Ipu=off  Pbase=100e6  Vbase=500e3  OutputType=Complex  PhasorSimulation=off  PSBequivalent=0
  To Workspace22 : ToWorkspace  VariableName=Vqd  SampleTime=-1
  To Workspace23 : ToWorkspace  VariableName=Iqd  SampleTime=-1
  V0 : Constant  Value=0
  Ain : PMIOPort  Side=Left
  Bin : PMIOPort  Port=2  Side=Left
  Cin : PMIOPort  Port=3  Side=Left
  Aout : PMIOPort  Port=4  Side=Right
  Bout : PMIOPort  Port=5  Side=Right
  Cout : PMIOPort  Port=6  Side=Right
  GND : PMIOPort  Port=7  Side=Left
  wires:
  Mux23/1 -> Inverse Park Transform/1(qd0)
  V0/1 -> Mux23/3
  Product/1 -> Demux1/1
  Demux1/1 -> Goto4/1
  Demux1/3 -> [C]
  Demux1/2 -> [B]
  Cos/1 -> Product1/2
  Constant21/1 -> Product1/1
  Product1/1 -> Mux23/1
  Cos1/1 -> Product2/1
  Integrator/1 -> Cos/1, Cos1/1
  Constant19/1 -> Integrator/1
  Product2/1 -> Mux23/2
  Constant18/1 -> Product2/2
  Mux2/1 -> To Workspace22/1
  [theta] -> Park Transform/2(wt)
  [Vabc5] -> Park Transform/1(ABC)
  Park Transform/1(qd0) -> Demux2/1
  Demux2/3 -> Terminator2/1
  theta/1 -> [theta]
  [theta] -> Inverse Park Transform/2(theta)
  Inverse Park Transform/1(ABC) -> Product/2
  Disturbance activator/1 -> Product/1
  Demux2/1 -> Mux2/1
  Demux2/2 -> Mux2/2
  Mux1/1 -> To Workspace23/1
  Demux3/3 -> Terminator1/1
  [Iabc5] -> Park Transform1/1(ABC)
  Park Transform1/1(qd0) -> Demux3/1
  Demux3/2 -> Mux1/2
  Demux3/1 -> Mux1/1
  [theta] -> Park Transform1/2(wt)
  From8/1 -> Controlled Current Source/1
  [C] -> Controlled Current Source2/1
  [B] -> Controlled Current Source1/1
  connections:
  Controlled Current Source1/LConn1 -- GND/RConn1 -- Controlled Current Source2/LConn1 -- Controlled Current Source/LConn1
  Ain/RConn1 -- Three-Phase V-I Measurement3/LConn1 -- Controlled Current Source/RConn1
  Bin/RConn1 -- Three-Phase V-I Measurement3/LConn2 -- Controlled Current Source1/RConn1
  Cin/RConn1 -- Three-Phase V-I Measurement3/LConn3 -- Controlled Current Source2/RConn1
  Three-Phase V-I Measurement3/RConn1 -- Aout/RConn1
  Three-Phase V-I Measurement3/RConn2 -- Bout/RConn1
  Three-Phase V-I Measurement3/RConn3 -- Cout/RConn1

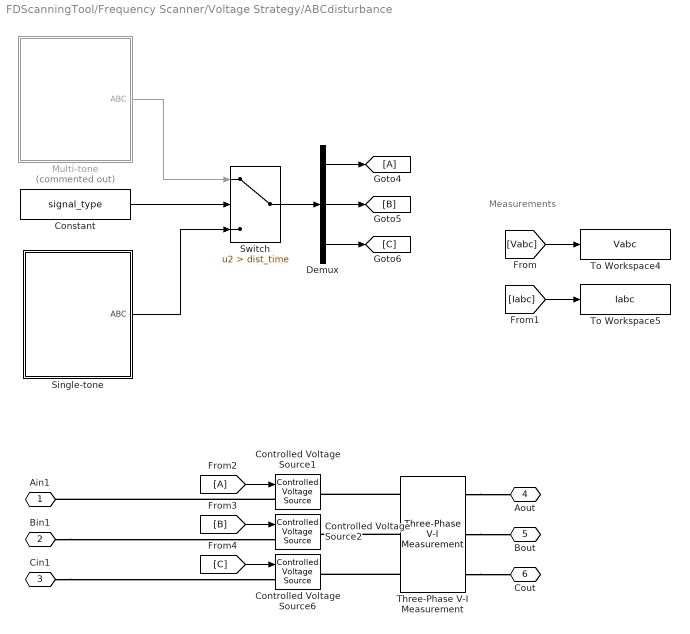
== system FDScanningTool/Frequency Scanner/Voltage Strategy/ABCdisturbance ==
  note: Measurements
  Constant : Constant  Value=signal_type
  Controlled Voltage Source1 : spsControlledVoltageSourceLib/Controlled Voltage Source  Initialize=off  Source_Type=DC  Amplitude=0  Phase=0  Frequency=0  Measurements=None
  Controlled Voltage Source2 : spsControlledVoltageSourceLib/Controlled Voltage Source  Initialize=off  Source_Type=DC  Amplitude=0  Phase=0  Frequency=0  Measurements=None
  Controlled Voltage Source6 : spsControlledVoltageSourceLib/Controlled Voltage Source  Initialize=off  Source_Type=DC  Amplitude=0  Phase=0  Frequency=0  Measurements=None
  Demux : Demux  Outputs=3
  From2 : From
  Goto4 : Goto
  Multi-tone : Subsystem  Commented=on
  Single-tone : Subsystem
  Switch : Switch  Criteria=u2 > Threshold  Threshold=dist_time  SaturateOnIntegerOverflow=off  InputSameDT=off
  Three-Phase V-I Measurement : spsThreePhaseVIMeasurementLib/Three-Phase V-I Measurement  VoltageMeasurement=phase-to-ground  SetLabelV=on  LabelV=Vabc  Vpu=off  VpuLL=off  CurrentMeasurement=yes  SetLabelI=on  LabelI=Iabc  Ipu=off  Pbase=100e6  Vbase=500e3  OutputType=Complex  PhasorSimulation=off  PSBequivalent=0
  To Workspace4 : ToWorkspace  VariableName=Vabc  SampleTime=-1
  To Workspace5 : ToWorkspace  VariableName=Iabc  SampleTime=-1
  Ain1 : PMIOPort  Side=Left
  Bin1 : PMIOPort  Port=2  Side=Left
  Cin1 : PMIOPort  Port=3  Side=Left
  Aout : PMIOPort  Port=4  Side=Right
  Bout : PMIOPort  Port=5  Side=Right
  Cout : PMIOPort  Port=6  Side=Right
  wires:
  [Vabc] -> To Workspace4/1
  [Iabc] -> To Workspace5/1
  [C] -> Controlled Voltage Source6/1
  From2/1 -> Controlled Voltage Source1/1
  [B] -> Controlled Voltage Source2/1
  Multi-tone/1(ABC) -> Switch/1
  Demux/3 -> [C]
  Constant/1 -> Switch/2
  Demux/1 -> Goto4/1
  Demux/2 -> [B]
  Single-tone/1(ABC) -> Switch/3
  Switch/1 -> Demux/1
  connections:
  Bin1/RConn1 -- Controlled Voltage Source2/LConn1
  Controlled Voltage Source1/LConn1 -- Ain1/RConn1
  Cin1/RConn1 -- Controlled Voltage Source6/LConn1
  Three-Phase V-I Measurement/LConn1 -- Controlled Voltage Source1/RConn1
  Three-Phase V-I Measurement/LConn2 -- Controlled Voltage Source2/RConn1
  Three-Phase V-I Measurement/LConn3 -- Controlled Voltage Source6/RConn1
  Three-Phase V-I Measurement/RConn3 -- Cout/RConn1
  Three-Phase V-I Measurement/RConn2 -- Bout/RConn1
  Three-Phase V-I Measurement/RConn1 -- Aout/RConn1

== system FDScanningTool/Frequency Scanner/Voltage Strategy/Voltage Fundamental Source ==
  Controlled Voltage Source1 : spsControlledVoltageSourceLib/Controlled Voltage Source  Initialize=off  Source_Type=DC  Amplitude=0  Phase=0  Frequency=0  Measurements=None
  Controlled Voltage Source2 : spsControlledVoltageSourceLib/Controlled Voltage Source  Initialize=off  Source_Type=DC  Amplitude=0  Phase=0  Frequency=0  Measurements=None
  Controlled Voltage Source3 : spsControlledVoltageSourceLib/Controlled Voltage Source  Initialize=off  Source_Type=DC  Amplitude=0  Phase=0  Frequency=0  Measurements=None
  Grid Voltages : Subsystem
  Ground : spsGroundLib/Ground  LConnTagsString=a
  Three-Phase Series RLC Branch : spsThreePhaseSeriesRLCBranchLib/Three-Phase Series RLC Branch  LConnTagsString=A|B|C  RConnTagsString=A|B|C  BranchType=R  Resistance=Rsource  Inductance=1e-3  Capacitance=1e-6  Measurements=None
  VzA : PMIOPort  Side=Right
  VzB : PMIOPort  Port=2  Side=Right
  VzC : PMIOPort  Port=3  Side=Right
  theta : Outport
  wires:
  Grid Voltages/3(VC) -> Controlled Voltage Source3/1
  Grid Voltages/2(VB) -> Controlled Voltage Source2/1
  Grid Voltages/1(VA) -> Controlled Voltage Source1/1
  Grid Voltages/4(theta) -> theta/1
  connections:
  Controlled Voltage Source2/LConn1 -- Controlled Voltage Source1/LConn1 -- Controlled Voltage Source3/LConn1 -- Ground/LConn1
  Three-Phase Series RLC Branch/RConn1 -- Controlled Voltage Source1/RConn1
  Three-Phase Series RLC Branch/RConn2 -- Controlled Voltage Source2/RConn1
  Three-Phase Series RLC Branch/RConn3 -- Controlled Voltage Source3/RConn1
  Three-Phase Series RLC Branch/LConn3 -- VzC/RConn1
  Three-Phase Series RLC Branch/LConn2 -- VzB/RConn1
  Three-Phase Series RLC Branch/LConn1 -- VzA/RConn1

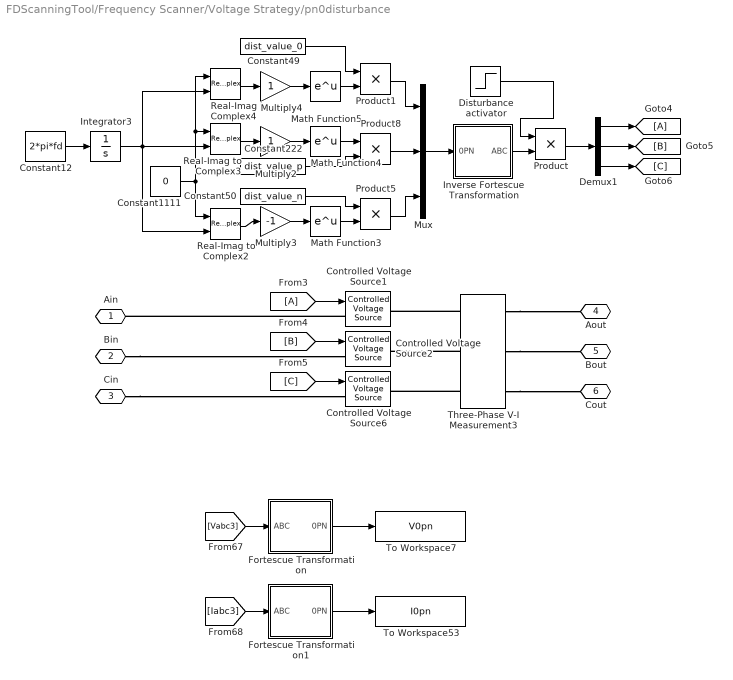
== system FDScanningTool/Frequency Scanner/Voltage Strategy/pn0disturbance ==
  Constant1111 : Constant  Value=0
  Constant12 : Constant  Value=2*pi*fd  SampleTime=delta_t
  Constant222 : Constant  Value=dist_value_p
  Constant49 : Constant  Value=dist_value_0
  Constant50 : Constant  Value=dist_value_n
  Controlled Voltage Source1 : spsControlledVoltageSourceLib/Controlled Voltage Source  Initialize=off  Source_Type=DC  Amplitude=0  Phase=0  Frequency=0  Measurements=None
  Controlled Voltage Source2 : spsControlledVoltageSourceLib/Controlled Voltage Source  Initialize=off  Source_Type=DC  Amplitude=0  Phase=0  Frequency=0  Measurements=None
  Controlled Voltage Source6 : spsControlledVoltageSourceLib/Controlled Voltage Source  Initialize=off  Source_Type=DC  Amplitude=0  Phase=0  Frequency=0  Measurements=None
  Demux1 : Demux  Outputs=3
  Disturbance activator : Step  Time=dist_time  SampleTime=delta_t
  Fortescue Transformation : Subsystem
  Fortescue Transformation1 : Subsystem
  From3 : From
  Goto4 : Goto
  Integrator3 : Integrator
  Inverse Fortescue Transformation : Subsystem
  Math Function3 : Math
  Math Function4 : Math
  Math Function5 : Math
  Multiply2 : Gain
  Multiply3 : Gain  Gain=-1
  Multiply4 : Gain
  Mux : Mux  Inputs=3
  Product{,1,5,8} (4 alike) : Product
  Real-Imag to Complex2 : RealImagToComplex
  Real-Imag to Complex3 : RealImagToComplex
  Real-Imag to Complex4 : RealImagToComplex
  Three-Phase V-I Measurement3 : spsThreePhaseVIMeasurementLib/Three-Phase V-I Measurement  VoltageMeasurement=phase-to-ground  SetLabelV=on  LabelV=Vabc3  Vpu=off  VpuLL=off  CurrentMeasurement=yes  SetLabelI=on  LabelI=Iabc3  Ipu=off  Pbase=100e6  Vbase=500e3  OutputType=Complex  PhasorSimulation=off  PSBequivalent=0
  To Workspace53 : ToWorkspace  VariableName=I0pn  SampleTime=-1
  To Workspace7 : ToWorkspace  VariableName=V0pn  SampleTime=-1
  Ain : PMIOPort  Side=Left
  Bin : PMIOPort  Port=2  Side=Left
  Cin : PMIOPort  Port=3  Side=Left
  Aout : PMIOPort  Port=4  Side=Right
  Bout : PMIOPort  Port=5  Side=Right
  Cout : PMIOPort  Port=6  Side=Right
  wires:
  Product/1 -> Demux1/1
  Demux1/1 -> Goto4/1
  Demux1/3 -> [C]
  Demux1/2 -> [B]
  Mux/1 -> Inverse Fortescue Transformation/1(0PN)
  Multiply2/1 -> Math Function4/1
  Integrator3/1 -> Real-Imag to Complex2/2, Real-Imag to Complex3/2, Real-Imag to Complex4/2
  Constant1111/1 -> Real-Imag to Complex4/1, Real-Imag to Complex3/1, Real-Imag to Complex2/1
  Real-Imag to Complex3/1 -> Multiply2/1
  Multiply3/1 -> Math Function3/1
  Constant12/1 -> Integrator3/1
  Real-Imag to Complex2/1 -> Multiply3/1
  Math Function5/1 -> Product1/2
  Real-Imag to Complex4/1 -> Multiply4/1
  Multiply4/1 -> Math Function5/1
  Product1/1 -> Mux/1
  [B] -> Controlled Voltage Source2/1
  From3/1 -> Controlled Voltage Source1/1
  [C] -> Controlled Voltage Source6/1
  Disturbance activator/1 -> Product/1
  Inverse Fortescue Transformation/1(ABC) -> Product/2
  Constant49/1 -> Product1/1
  Math Function3/1 -> Product5/2
  Constant50/1 -> Product5/1
  Math Function4/1 -> Product8/1
  Constant222/1 -> Product8/2
  Product8/1 -> Mux/2
  Product5/1 -> Mux/3
  [Vabc3] -> Fortescue Transformation/1(ABC)
  [Iabc3] -> Fortescue Transformation1/1(ABC)
  Fortescue Transformation/1(0PN) -> To Workspace7/1
  Fortescue Transformation1/1(0PN) -> To Workspace53/1
  connections:
  Controlled Voltage Source1/LConn1 -- Ain/RConn1
  Cin/RConn1 -- Controlled Voltage Source6/LConn1
  Bin/RConn1 -- Controlled Voltage Source2/LConn1
  Three-Phase V-I Measurement3/LConn1 -- Controlled Voltage Source1/RConn1
  Three-Phase V-I Measurement3/LConn2 -- Controlled Voltage Source2/RConn1
  Three-Phase V-I Measurement3/LConn3 -- Controlled Voltage Source6/RConn1
  Three-Phase V-I Measurement3/RConn1 -- Aout/RConn1
  Three-Phase V-I Measurement3/RConn2 -- Bout/RConn1
  Three-Phase V-I Measurement3/RConn3 -- Cout/RConn1

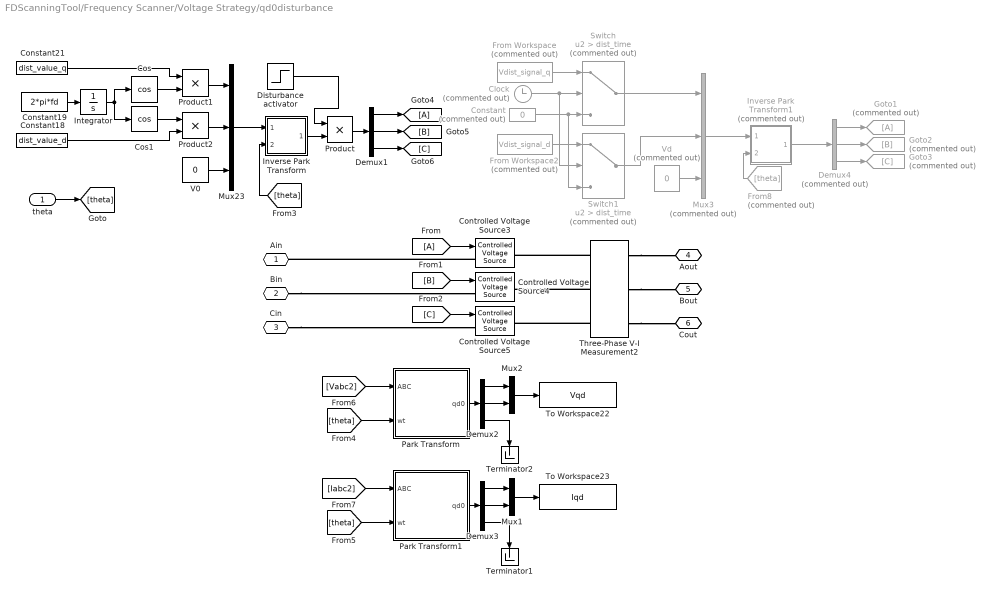
== system FDScanningTool/Frequency Scanner/Voltage Strategy/qd0disturbance ==
  theta : Inport
  Clock : Clock  Commented=on
  Constant : Constant  Commented=on  Value=0
  Constant18 : Constant  Value=dist_value_d
  Constant19 : Constant  Value=2*pi*fd
  Constant21 : Constant  Value=dist_value_q
  Controlled Voltage Source3 : spsControlledVoltageSourceLib/Controlled Voltage Source  Initialize=off  Source_Type=DC  Amplitude=0  Phase=0  Frequency=0  Measurements=None
  Controlled Voltage Source4 : spsControlledVoltageSourceLib/Controlled Voltage Source  Initialize=off  Source_Type=DC  Amplitude=0  Phase=0  Frequency=0  Measurements=None
  Controlled Voltage Source5 : spsControlledVoltageSourceLib/Controlled Voltage Source  Initialize=off  Source_Type=DC  Amplitude=0  Phase=0  Frequency=0  Measurements=None
  Cos : Trigonometry  Operator=cos
  Cos1 : Trigonometry  Operator=cos
  Demux1 : Demux  Outputs=3
  Demux2 : Demux  Outputs=3
  Demux3 : Demux  Outputs=3
  Demux4 : Demux  Commented=on  Outputs=3
  Disturbance activator : Step  Time=dist_time  Before=0.0  After=1.0  SampleTime=delta_t
  From : From
  From Workspace : FromWorkspace  Commented=on  VariableName=Vdist_signal_q  SampleTime=delta_t
  From Workspace2 : FromWorkspace  Commented=on  VariableName=Vdist_signal_d  SampleTime=delta_t
  From8 : From  Commented=on  GotoTag=theta
  Goto1 : Goto  Commented=on
  Goto2 : Goto  Commented=on  GotoTag=B
  Goto3 : Goto  Commented=on  GotoTag=C
  Goto4 : Goto
  Integrator : Integrator
  Inverse Park Transform : Subsystem
  Inverse Park Transform1 : Subsystem  Commented=on
  Mux1 : Mux  Inputs=2
  Mux2 : Mux  Inputs=2
  Mux23 : Mux  Inputs=3
  Mux3 : Mux  Commented=on  Inputs=3
  Park Transform : Subsystem
  Park Transform1 : Subsystem
  Product : Product
  Product1 : Product
  Product2 : Product
  Switch : Switch  Commented=on  Criteria=u2 > Threshold  Threshold=dist_time  SaturateOnIntegerOverflow=off  InputSameDT=off
  Switch1 : Switch  Commented=on  Criteria=u2 > Threshold  Threshold=dist_time  SaturateOnIntegerOverflow=off  InputSameDT=off
  Terminator1 : Terminator
  Terminator2 : Terminator
  Three-Phase V-I Measurement2 : spsThreePhaseVIMeasurementLib/Three-Phase V-I Measurement  VoltageMeasurement=phase-to-ground  SetLabelV=on  LabelV=Vabc2  Vpu=off  VpuLL=off  CurrentMeasurement=yes  SetLabelI=on  LabelI=Iabc2  Ipu=off  Pbase=100e6  Vbase=500e3  OutputType=Complex  PhasorSimulation=off  PSBequivalent=0
  To Workspace22 : ToWorkspace  VariableName=Vqd  SampleTime=-1
  To Workspace23 : ToWorkspace  VariableName=Iqd  SampleTime=-1
  V0 : Constant  Value=0
  Vd : Constant  Commented=on  Value=0
  Ain : PMIOPort  Side=Left
  Bin : PMIOPort  Port=2  Side=Left
  Cin : PMIOPort  Port=3  Side=Left
  Aout : PMIOPort  Port=4  Side=Right
  Bout : PMIOPort  Port=5  Side=Right
  Cout : PMIOPort  Port=6  Side=Right
  wires:
  Mux23/1 -> Inverse Park Transform/1(qd0)
  V0/1 -> Mux23/3
  From/1 -> Controlled Voltage Source3/1
  [B] -> Controlled Voltage Source4/1
  [C] -> Controlled Voltage Source5/1
  Product/1 -> Demux1/1
  Demux1/1 -> Goto4/1
  Demux1/3 -> [C]
  Demux1/2 -> [B]
  Cos/1 -> Product1/2
  Constant21/1 -> Product1/1
  Product1/1 -> Mux23/1
  Cos1/1 -> Product2/1
  Integrator/1 -> Cos/1, Cos1/1
  Constant19/1 -> Integrator/1
  Product2/1 -> Mux23/2
  Constant18/1 -> Product2/2
  Mux2/1 -> To Workspace22/1
  [theta] -> Park Transform/2(wt)
  [Vabc2] -> Park Transform/1(ABC)
  Park Transform/1(qd0) -> Demux2/1
  Demux2/3 -> Terminator2/1
  theta/1 -> [theta]
  [theta] -> Inverse Park Transform/2(theta)
  Inverse Park Transform/1(ABC) -> Product/2
  Disturbance activator/1 -> Product/1
  Demux2/1 -> Mux2/1
  Demux2/2 -> Mux2/2
  Mux1/1 -> To Workspace23/1
  Demux3/3 -> Terminator1/1
  [Iabc2] -> Park Transform1/1(ABC)
  Park Transform1/1(qd0) -> Demux3/1
  Demux3/2 -> Mux1/2
  Demux3/1 -> Mux1/1
  [theta] -> Park Transform1/2(wt)
  From Workspace/1 -> Switch/1
  Clock/1 -> Switch/2, Switch1/2
  From Workspace2/1 -> Switch1/1
  Constant/1 -> Switch1/3, Switch/3
  Switch/1 -> Mux3/1
  Switch1/1 -> Mux3/2
  Vd/1 -> Mux3/3
  Mux3/1 -> Inverse Park Transform1/1(qd0)
  From8/1 -> Inverse Park Transform1/2(theta)
  Inverse Park Transform1/1(ABC) -> Demux4/1
  Demux4/3 -> Goto3/1
  Demux4/2 -> Goto2/1
  Demux4/1 -> Goto1/1
  connections:
  Controlled Voltage Source3/LConn1 -- Ain/RConn1
  Bin/RConn1 -- Controlled Voltage Source4/LConn1
  Cin/RConn1 -- Controlled Voltage Source5/LConn1
  Three-Phase V-I Measurement2/LConn1 -- Controlled Voltage Source3/RConn1
  Three-Phase V-I Measurement2/LConn2 -- Controlled Voltage Source4/RConn1
  Three-Phase V-I Measurement2/LConn3 -- Controlled Voltage Source5/RConn1
  Three-Phase V-I Measurement2/RConn1 -- Aout/RConn1
  Three-Phase V-I Measurement2/RConn2 -- Bout/RConn1
  Three-Phase V-I Measurement2/RConn3 -- Cout/RConn1

== system FDScanningTool/Frequency Scanner/Current Strategy/ABCdisturbance2/Multi-tone ==
  Clock : Clock
  Constant1 : Constant  Value=0
  From Workspace : FromWorkspace  VariableName=dist_value_a  SampleTime=delta_t
  From Workspace1 : FromWorkspace  VariableName=dist_value_b  SampleTime=delta_t
  From Workspace2 : FromWorkspace  VariableName=dist_value_c  SampleTime=delta_t
  Mux : Mux  Inputs=3
  Switch1 : Switch  Criteria=u2 > Threshold  Threshold=dist_time  SaturateOnIntegerOverflow=off  InputSameDT=off
  Switch2 : Switch  Criteria=u2 > Threshold  Threshold=dist_time  SaturateOnIntegerOverflow=off  InputSameDT=off
  Switch3 : Switch  Criteria=u2 > Threshold  Threshold=dist_time  SaturateOnIntegerOverflow=off  InputSameDT=off
  ABC : Outport
  wires:
  Switch2/1 -> Mux/2
  From Workspace2/1 -> Switch3/1
  Constant1/1 -> Switch3/3, Switch2/3, Switch1/3
  From Workspace1/1 -> Switch2/1
  Switch3/1 -> Mux/3
  Clock/1 -> Switch1/2, Switch2/2, Switch3/2
  Switch1/1 -> Mux/1
  From Workspace/1 -> Switch1/1
  Mux/1 -> ABC/1

== system FDScanningTool/Frequency Scanner/Current Strategy/ABCdisturbance2/Single-tone ==
  note: ABC perturbance
  Constant10 : Constant  Value=phi
  Constant12 : Constant  Value=2*pi*fd  SampleTime=delta_t
  Constant9 : Constant  Value=phi
  Integrator5 : Integrator  UpperSaturationLimit=1E100  LowerSaturationLimit=-1E100
  Mux : Mux  Inputs=3
  Product1 : Product
  Product2 : Product
  Product3 : Product
  Sin : Trigonometry  Operator=cos
  Sin1 : Trigonometry  Operator=cos
  Sin2 : Trigonometry  Operator=cos
  Step1 : Step  Time=dist_time  After=dist_value_a  SampleTime=delta_t
  Step2 : Step  Time=dist_time  After=dist_value_b  SampleTime=delta_t
  Step3 : Step  Time=dist_time  After=dist_value_c  SampleTime=delta_t
  Sum6 : Sum  Inputs=|+-
  Sum7 : Sum  Inputs=|++
  ABC : Outport
  wires:
  Sin/1 -> Product1/1
  Sum7/1 -> Sin2/1
  Product1/1 -> Mux/1
  Integrator5/1 -> Sum7/1, Sin/1, Sum6/1
  Sin1/1 -> Product2/1
  Sin2/1 -> Product3/1
  Constant9/1 -> Sum6/2
  Constant10/1 -> Sum7/2
  Step3/1 -> Product3/2
  Step2/1 -> Product2/2
  Constant12/1 -> Integrator5/1
  Sum6/1 -> Sin1/1
  Step1/1 -> Product1/2
  Product2/1 -> Mux/2
  Product3/1 -> Mux/3
  Mux/1 -> ABC/1
